simulink model "quarter_car_model"  (R2024a)
settings: Solver=VariableStepAuto  StartTime=0.0  StopTime=endtime  RelTol=1e-3
undefined symbols (not defined in the file): A, Aa, B, Ba, C, Ca, D, Da, input_signal, Kd, Ki, Kp, noise_enabled, sat
libraries: simulink x3, slpidlib x1, dspstat3 x1
settings Model: Creator=moham  LastModifiedBy=moham

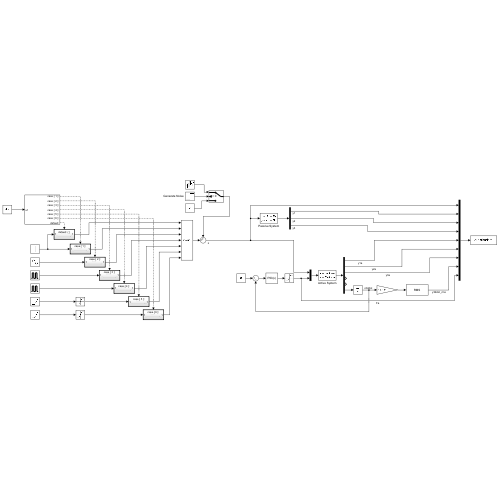
[thumbnail: Simulink's stored preview of the top-level diagram]
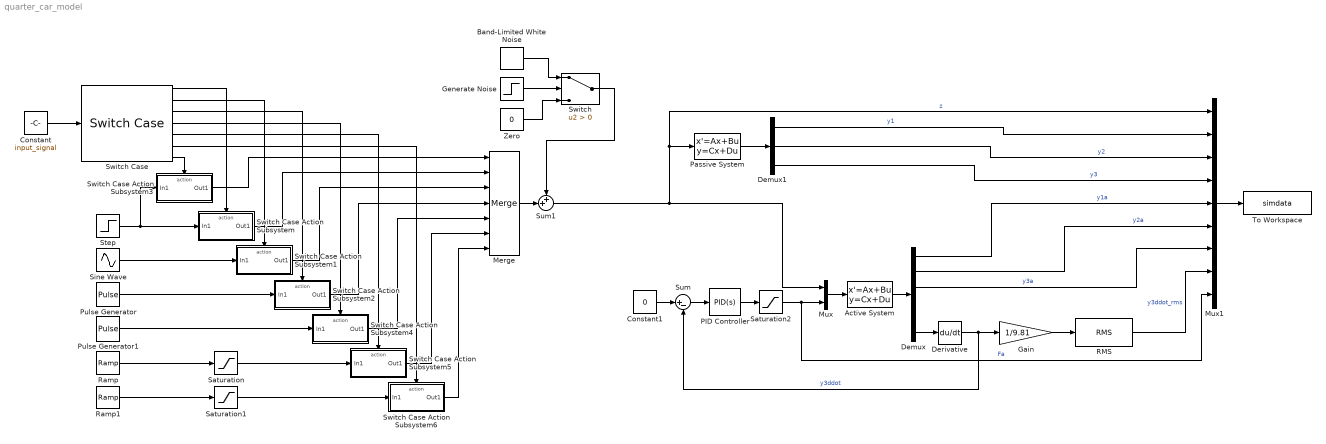
== system quarter_car_model ==
  Active System : StateSpace  A=Aa  B=Ba  C=Ca  D=Da  InitialCondition=0
  Band-Limited White Noise : simulink/Sources/Band-Limited White Noise  Cov=[0.0000001]  Ts=0.01  seed=[23341]
  Constant : Constant  Value=input_signal
  Constant1 : Constant  Value=0
  Demux : Demux  Outputs=6
  Demux1 : Demux  Outputs=3
  Derivative : Derivative
  Gain : Gain  Gain=1/9.81
  Generate Noise : Step  Time=0  After=noise_enabled  SampleTime=0
  Merge : Merge  Inputs=7
  Mux : Mux  Inputs=2
  Mux1 : Mux  Inputs=9
  PID Controller : slpidlib/PID Controller  Controller=PID  Form=Parallel  TimeDomain=Continuous-time  UseExternalTs=off  SampleTime=-1  IntegratorMethod=Forward Euler  FilterMethod=Forward Euler  ControllerParametersSource=internal  P=Kp  I=Ki  UseKiTs=off  D=Kd  UseExternalDerivativeSource=off  N=2.78597764038136  UseFilter=on  TunerSelectOption=Transfer Function Based (PID Tuner App)  InitialConditionSource=internal  InitialConditionForIntegrator=0  InitialConditionForFilter=0  DifferentiatorICPrevScaledInput=0  ExternalReset=none  TrackingMode=off  Kt=1  LimitOutput=off  SatLimitsSource=internal  UpperSaturationLimit=inf  LowerSaturationLimit=-inf  LinearizeAsGain=on  AntiWindupMode=none  Kb=1  LimitIntegrator=off  UpperIntegratorSaturationLimit=inf  LowerIntegratorSaturationLimit=-inf  POutMin=[]  POutMax=[]  IOutMin=[]  IOutMax=[]  DOutMin=[]  DOutMax=[]  NOutMin=[]  NOutMax=[]  SumOutMin=[]  SumOutMax=[]  SaturationOutMin=[]  SaturationOutMax=[]  PParamMin=[]  PParamMax=[]  IParamMin=[]  IParamMax=[]  DParamMin=[]  DParamMax=[]  NParamMin=[]  NParamMax=[]  KbParamMin=[]  KbParamMax=[]  KtParamMin=[]  KtParamMax=[]  KbOutMin=[]  KbOutMax=[]  KtOutMin=[]  KtOutMax=[]  IntegratorOutMin=[]  IntegratorOutMax=[]  FilterOutMin=[]  FilterOutMax=[]  SumI1OutMin=[]  SumI1OutMax=[]  SumI2OutMin=[]  SumI2OutMax=[]  SumI3OutMin=[]  SumI3OutMax=[]  SumI4OutMin=[]  SumI4OutMax=[]  SumDOutMin=[]  SumDOutMax=[]  DifferentiatorOutMin=[]  DifferentiatorOutMax=[]  FilterDiffOutCoefMin=[]  FilterDiffOutCoefMax=[]  ReciprocalOutMin=[]  ReciprocalOutMax=[]  SumDenOutMin=[]  SumDenOutMax=[]  SumNumOutMin=[]  SumNumOutMax=[]  DivideOutMin=[]  DivideOutMax=[]  UdiffTsProdOutMin=[]  UdiffTsProdOutMax=[]  NTsProdOutMin=[]  NTsProdOutMax=[]  UintegralTsProdOutMin=[]  UintegralTsProdOutMax=[]  UngainTsProdOutMin=[]  UngainTsProdOutMax=[]  ClampingZeroOutDataTypeStr=Inherit: Inherit via back propagation  ClampingZeroOutMin=[]  ClampingZeroOutMax=[]  FilterDenConstantOutDataTypeStr=Inherit: Inherit via back propagation  FilterDenConstantOutMin=[]  FilterDenConstantOutMax=[]  PCopyOutDataTypeStr=Inherit: Inherit via back propagation  PCopyOutMin=[]  PCopyOutMax=[]  NCopyOutDataTypeStr=Inherit: Inherit via back propagation  NCopyOutMin=[]  NCopyOutMax=[]  IntegratorContinuousStateAttributes=''  IntegratorStateMustResolveToSignalObject=off  IntegratorRTWStateStorageClass=Auto  FilterContinuousStateAttributes=''  FilterStateMustResolveToSignalObject=off  FilterRTWStateStorageClass=Auto  ParallelPVariant=InternalParameters  IdealPVariant=Disabled  IVariant=InternalParameters  DVariant=InternalParameters  IntegratorVariant=Continuous  SatVariant=Disabled  AWVariant=Passthrough  PCopyVariant=Disabled  TRVariant=Disabled  FdbkBlocksVariant=Forward  IdealPFdbkVariant=Disabled  SatFdbkVariant=Disabled  DerivativeFilterVariant=ContFilter  NVariant=InternalParameters  NCopyVariant=Disabled  FilterICVariant=InternalICsFilter  IntegratorICVariant=InternalICs  ExternalResetVariant=Disabled  TRSumVariant=Passthrough  SumFdbkVariant=Disabled  SumVariant=Sum_PID  TsampFilterVariant=InternalTs  TsampNgainVariant=Passthrough  TsampIntegralVariant=Disabled_SignalSpec  ExternalSaturationOutDataTypeStr=Inherit: Same as second input  DerivativeSourceVariant=ErrorSignal
  Passive System : StateSpace  A=A  B=B  C=C  D=D  InitialCondition=0
  Pulse Generator : DiscretePulseGenerator  PulseType=Time based  Amplitude=0.1  Period=8  PulseWidth=5  PhaseDelay=2
  Pulse Generator1 : DiscretePulseGenerator  PulseType=Time based  Amplitude=-0.08  Period=8  PulseWidth=10  PhaseDelay=2
  RMS : dspstat3/RMS  run=off  directionMode=Entire input  dimension=1  InputProcessing=Columns as channels (frame based)  reset_popup=None
  Ramp : simulink/Sources/Ramp  slope=0.15  start=1  InitialOutput=0
  Ramp1 : simulink/Sources/Ramp  slope=-0.15  start=1  InitialOutput=0
  Saturation : Saturate  UpperLimit=2  LowerLimit=-2
  Saturation1 : Saturate  UpperLimit=2  LowerLimit=-2
  Saturation2 : Saturate  UpperLimit=sat  LowerLimit=-sat
  Sine Wave : Sin  Amplitude=0.15  SampleTime=0
  Step : Step  SampleTime=0
  Sum : Sum  Inputs=|+-
  Sum1 : Sum  Inputs=++|
  Switch : Switch  Criteria=u2 > Threshold  SaturateOnIntegerOverflow=off  InputSameDT=off
  Switch Case : SwitchCase  CaseConditions={1, 2, 3, 4, 5, 6}
  Switch Case Action Subsystem : Subsystem  TreatAsAtomicUnit=on
  Switch Case Action Subsystem1 : Subsystem  TreatAsAtomicUnit=on
  Switch Case Action Subsystem2 : Subsystem  TreatAsAtomicUnit=on
  Switch Case Action Subsystem3 : Subsystem  TreatAsAtomicUnit=on
  Switch Case Action Subsystem4 : Subsystem  TreatAsAtomicUnit=on
  Switch Case Action Subsystem5 : Subsystem  TreatAsAtomicUnit=on
  Switch Case Action Subsystem6 : Subsystem  TreatAsAtomicUnit=on
  To Workspace : ToWorkspace  VariableName=simdata  SaveFormat=Structure With Time  SampleTime=-1
  Zero : Constant  Value=0  OutDataTypeStr=Inherit: Inherit via back propagation
  wires:
  Passive System/1 -> Demux1/1
  Band-Limited White Noise/1 -> Switch/1
  Zero/1 -> Switch/3
  Generate Noise/1 -> Switch/2
  Step/1 -> Switch Case Action Subsystem3/1(In1), Switch Case Action Subsystem/1(In1)
  Switch Case/1 -> Switch Case Action Subsystem/Action
  Switch Case/2 -> Switch Case Action Subsystem1/Action
  Switch Case/3 -> Switch Case Action Subsystem2/Action
  Sine Wave/1 -> Switch Case Action Subsystem1/1(In1)
  Pulse Generator/1 -> Switch Case Action Subsystem2/1(In1)
  Switch Case/7 -> Switch Case Action Subsystem3/Action
  Switch/1 -> Sum1/1
  Sum1/1 -> Mux/1, Mux1/1, Passive System/1  "z"
  Constant/1 -> Switch Case/1
  Switch Case/4 -> Switch Case Action Subsystem4/Action
  Switch Case/5 -> Switch Case Action Subsystem5/Action
  Switch Case/6 -> Switch Case Action Subsystem6/Action
  Pulse Generator1/1 -> Switch Case Action Subsystem4/1(In1)
  Ramp/1 -> Saturation/1
  Ramp1/1 -> Saturation1/1
  Merge/1 -> Sum1/2
  Switch Case Action Subsystem3/1(Out1) -> Merge/1
  Switch Case Action Subsystem/1(Out1) -> Merge/2
  Switch Case Action Subsystem1/1(Out1) -> Merge/3
  Switch Case Action Subsystem2/1(Out1) -> Merge/4
  Switch Case Action Subsystem4/1(Out1) -> Merge/5
  Switch Case Action Subsystem5/1(Out1) -> Merge/6
  Switch Case Action Subsystem6/1(Out1) -> Merge/7
  Saturation/1 -> Switch Case Action Subsystem5/1(In1)
  Saturation1/1 -> Switch Case Action Subsystem6/1(In1)
  Mux/1 -> Active System/1
  PID Controller/1 -> Saturation2/1
  Saturation2/1 -> Mux/2, Mux1/9  "Fa"
  Active System/1 -> Demux/1
  Demux/6 -> Derivative/1
  Derivative/1 -> Sum/2, Gain/1  "y3ddot"
  Gain/1 -> RMS/1
  Mux1/1 -> To Workspace/1
  Demux1/1 -> Mux1/2  "y1"
  Demux1/2 -> Mux1/3  "y2"
  Demux1/3 -> Mux1/4  "y3"
  Demux/1 -> Mux1/5  "y1a"
  Demux/2 -> Mux1/6  "y2a"
  Demux/3 -> Mux1/7  "y3a"
  RMS/1 -> Mux1/8  "y3ddot_rms"
  Sum/1 -> PID Controller/1
  Constant1/1 -> Sum/1

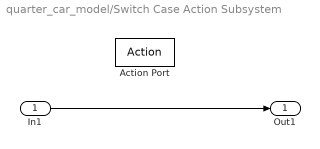
== system quarter_car_model/Switch Case Action Subsystem ==
  In1 : Inport
  Action Port : ActionPort  ActionPortLabel=case [ 1 ]:
  Out1 : Outport
  wires:
  In1/1 -> Out1/1

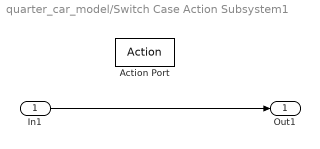
== system quarter_car_model/Switch Case Action Subsystem1 ==
  In1 : Inport
  Action Port : ActionPort  ActionPortLabel=case [ 2 ]:
  Out1 : Outport
  wires:
  In1/1 -> Out1/1

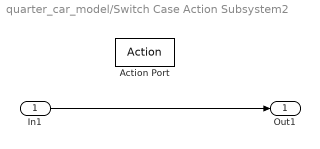
== system quarter_car_model/Switch Case Action Subsystem2 ==
  In1 : Inport
  Action Port : ActionPort  ActionPortLabel=case [ 3 ]:
  Out1 : Outport
  wires:
  In1/1 -> Out1/1

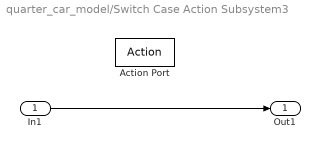
== system quarter_car_model/Switch Case Action Subsystem3 ==
  In1 : Inport
  Action Port : ActionPort  ActionPortLabel=default:
  Out1 : Outport
  wires:
  In1/1 -> Out1/1

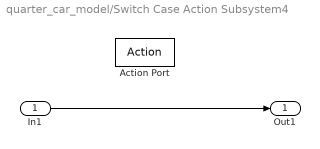
== system quarter_car_model/Switch Case Action Subsystem4 ==
  In1 : Inport
  Action Port : ActionPort  ActionPortLabel=case [ 4 ]:
  Out1 : Outport
  wires:
  In1/1 -> Out1/1

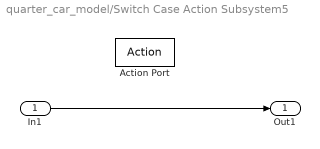
== system quarter_car_model/Switch Case Action Subsystem5 ==
  In1 : Inport
  Action Port : ActionPort  ActionPortLabel=case [ 5 ]:
  Out1 : Outport
  wires:
  In1/1 -> Out1/1

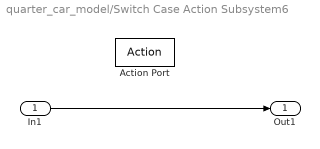
== system quarter_car_model/Switch Case Action Subsystem6 ==
  In1 : Inport
  Action Port : ActionPort  ActionPortLabel=case [ 6 ]:
  Out1 : Outport
  wires:
  In1/1 -> Out1/1
